simulink model "Lab1"  (R2022b)
settings: Solver=ode45  StartTime=0.0  StopTime=20  RelTol=1e-3
undefined symbols (not defined in the file): T, unicycle
libraries: simulink x2
settings Model: Creator=Musta  LastModifiedBy=Musta

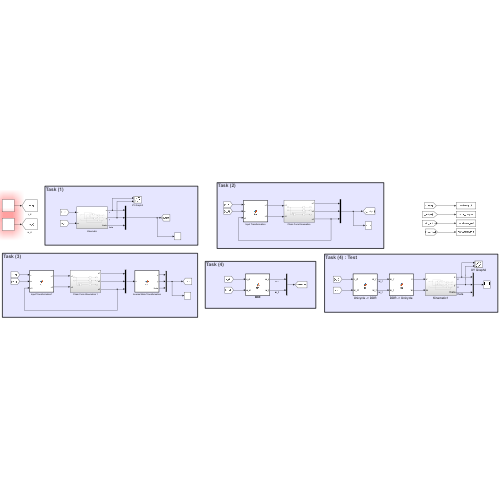
[thumbnail: Simulink's stored preview of the top-level diagram]
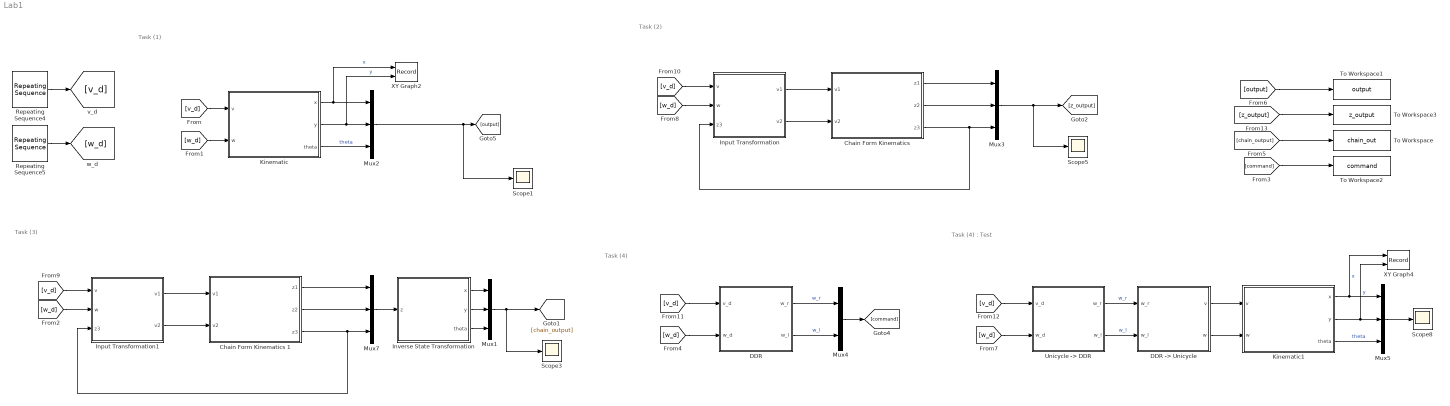
== system Lab1 ==
  note: Task (4) : Test
  note: Task (4)
  note: Task (2)
  note: Task (1)
  note: Task (3)
  " DDR -> Unicycle " : MATLAB Function  TreatAsAtomicUnit=on
  "Chain Form Kinematics " : Subsystem
  Chain Form Kinematics 1 : Subsystem
  DDR : MATLAB Function  TreatAsAtomicUnit=on
  Input Transformation : MATLAB Function  TreatAsAtomicUnit=on
  Input Transformation1 : MATLAB Function  TreatAsAtomicUnit=on
  Inverse State Transformation : MATLAB Function  TreatAsAtomicUnit=on
  Kinematic : Subsystem
  Kinematic1 : Subsystem
  Mux{1..3,5,7} (5 alike) : Mux  Inputs=3
  Mux4 : Mux  Inputs=2
  Repeating Sequence4 : simulink/Sources/Repeating Sequence  rep_seq_t=[0 T/3 2*T/3 T]  rep_seq_y=[0.1 0.1 0.3 0.05]
  Repeating Sequence5 : simulink/Sources/Repeating Sequence  rep_seq_t=[0 T/4 2*T/4 3*T/4 T]  rep_seq_y=[0.0 0.0 0.1 -0.1 0.15]
  Scope{1,3,5,8} (4 alike) : Scope
  To Workspace : ToWorkspace  VariableName=chain_out  SaveFormat=Structure With Time  SampleTime=-1
  To Workspace1 : ToWorkspace  VariableName=output  SaveFormat=Timeseries  SampleTime=-1
  To Workspace2 : ToWorkspace  VariableName=command  SaveFormat=Structure With Time  SampleTime=-1
  To Workspace3 : ToWorkspace  VariableName=z_output  SaveFormat=Structure With Time  SampleTime=-1
  "Unicycle -> DDR" : MATLAB Function  TreatAsAtomicUnit=on
  XY Graph2 : Record  FileSettingsInternal="{\"entries\":[{\"content\":{\"excelSettings\":{\"content\":{},\"type\":\"Streamout.ExcelSettings\"}},\"type\":\"Streamout.FileSettingStorage\",\"uuid\":\"3bdbee54-c759-43d2-8827-5e9ea4f4a11d\"}],\"packageUris\":[\"http://schema.mathworks.com/mf0/streamout_blocks/R2020a\"],\"version\":\"1.0\"}"  Layout=[1 1]  SignalsInternal="{\"entries\":[{\"content\":{\"signals\":[{\"content\":{\"blockPath\":[\"Lab1/XY Graph2\"],\"channel\":[],\"dimensions\":[1],\"domain\":\"Lab1/XY Graph2\",\"lineColor\":\"#a2142f\",\"plots\":[1],\"port\":1,\"sid\":[],\"signalID\":34,\"signalName\":\"x\"},\"type\":\"RecordBlkView.Signal\",\"uuid\":\"4d3c6372-cd81-4779-b9ee-b57c7a1f23b0\"},{\"content\":{\"blockPath\":[\"Lab1/XY Graph2\"],\"channel\":[],\"dimensions\":[1],\"domain\":\"Lab1/XY Graph2\",\"lineColor\":\"#139fff\",\"plots\":[1],\"port\":2,\"sid\":[],\"signalID\":37,\"signalName\":\"y\"},\"type\":\"RecordBlkView.Signal\",\"uuid\":\"7a674121-f9e3-4504-b1cd-7ca841214a66\"}]},\"type\":\"RecordBlkView.InputSignals\",\"uuid\":\"66f41a1e-2d26-4257-ac1b-8d37125b5a9b\"}],\"packageUris\":[\"http://schema.mathworks.com/mf0/streamout_blocks/R2020a\"],\"version\":\"1.0\"}"  VisualizationBindings="{\"xyplotplugin\":{\"info\":[{\"series\":[{\"bindingParametersList\":[{\"parameter\":\"X-Axis\",\"signalID\":34,\"signalName\":\"x\"},{\"parameter\":\"Y-Axis\",\"signalID\":37,\"signalName\":\"y\"}],\"seriesID\":44568}],\"subplotID\":1}]}}"  CompatibilityTag=XY
  XY Graph4 : Record  FileSettingsInternal="{\"entries\":[{\"content\":{\"excelSettings\":{\"content\":{},\"type\":\"Streamout.ExcelSettings\"}},\"type\":\"Streamout.FileSettingStorage\",\"uuid\":\"aad4d6af-3abc-44fb-a7f4-f6db2a127860\"}],\"packageUris\":[\"http://schema.mathworks.com/mf0/streamout_blocks/R2020a\"],\"version\":\"1.0\"}"  Layout=[1 1]  SignalsInternal="{\"entries\":[{\"content\":{\"signals\":[{\"content\":{\"blockPath\":[\"Lab1/XY Graph4\"],\"channel\":[],\"dimensions\":[1],\"domain\":\"Lab1/XY Graph4\",\"lineColor\":\"#a2142f\",\"plots\":[1],\"port\":1,\"sid\":[],\"signalID\":26,\"signalName\":\"x\"},\"type\":\"RecordBlkView.Signal\",\"uuid\":\"5aadf423-cf44-42bb-a75c-07b2a2665d40\"},{\"content\":{\"blockPath\":[\"Lab1/XY Graph4\"],\"channel\":[],\"dimensions\":[1],\"domain\":\"Lab1/XY Graph4\",\"lineColor\":\"#139fff\",\"plots\":[1],\"port\":2,\"sid\":[],\"signalID\":29,\"signalName\":\"y\"},\"type\":\"RecordBlkView.Signal\",\"uuid\":\"69a4f6a6-7bec-4189-9cf2-ac6d9897c812\"}]},\"type\":\"RecordBlkView.InputSignals\",\"uuid\":\"eab3d5d4-c8e6-4073-8c70-e7f334e51194\"}],\"packageUris\":[\"http://schema.mathworks.com/mf0/streamout_blocks/R2020a\"],\"version\":\"1.0\"}"  VisualizationBindings="{\"xyplotplugin\":{\"info\":[{\"series\":[{\"bindingParametersList\":[{\"parameter\":\"X-Axis\",\"signalID\":26,\"signalName\":\"x\"},{\"parameter\":\"Y-Axis\",\"signalID\":29,\"signalName\":\"y\"}],\"seriesID\":23320}],\"subplotID\":1}]}}"  CompatibilityTag=XY
  wires:
  Repeating Sequence4/1 -> [v_d]
  Repeating Sequence5/1 -> [w_d]
  [w_d] -> DDR/2(w_d)
  "Unicycle -> DDR"/2(w_l) -> " DDR -> Unicycle "/2(w_l)  "w_l"
  Input Transformation1/2(v2) -> Chain Form Kinematics 1/2(v2)
  Input Transformation/1(v1) -> "Chain Form Kinematics "/1(v1)
  [w_d] -> "Unicycle -> DDR"/2(w_d)
  Input Transformation1/1(v1) -> Chain Form Kinematics 1/1(v1)
  Chain Form Kinematics 1/2(z2) -> Mux7/2
  [v_d] -> DDR/1(v_d)
  Kinematic1/2(y) -> Mux5/2, XY Graph4/2  "y"
  "Chain Form Kinematics "/2(z2) -> Mux3/2
  "Unicycle -> DDR"/1(w_r) -> " DDR -> Unicycle "/1(w_r)  "w_r"
  Kinematic/3(theta) -> Mux2/3  "theta"
  DDR/2(w_l) -> Mux4/2  "w_l"
  [w_d] -> Input Transformation1/2(w)
  [v_d] -> Input Transformation1/1(v)
  Chain Form Kinematics 1/1(z1) -> Mux7/1
  Kinematic1/1(x) -> Mux5/1, XY Graph4/1  "x"
  Mux5/1 -> Scope8/1
  " DDR -> Unicycle "/1(v) -> Kinematic1/1(v)
  Kinematic1/3(theta) -> Mux5/3  "theta"
  Kinematic/1(x) -> Mux2/1, XY Graph2/1  "x"
  "Chain Form Kinematics "/1(z1) -> Mux3/1
  Kinematic/2(y) -> Mux2/2, XY Graph2/2  "y"
  Chain Form Kinematics 1/3(z3) -> Mux7/3, Input Transformation1/3(z3)
  Input Transformation/2(v2) -> "Chain Form Kinematics "/2(v2)
  [w_d] -> Kinematic/2(w)
  " DDR -> Unicycle "/2(w) -> Kinematic1/2(w)
  Mux3/1 -> [z_output], Scope5/1
  [v_d] -> "Unicycle -> DDR"/1(v_d)
  [v_d] -> Kinematic/1(v)
  Mux7/1 -> Inverse State Transformation/1(z)
  [v_d] -> Input Transformation/1(v)
  [w_d] -> Input Transformation/2(w)
  "Chain Form Kinematics "/3(z3) -> Mux3/3, Input Transformation/3(z3)
  Inverse State Transformation/2(y) -> Mux1/2
  Inverse State Transformation/3(theta) -> Mux1/3
  Mux1/1 -> [chain_output], Scope3/1
  Inverse State Transformation/1(x) -> Mux1/1
  [output] -> To Workspace1/1
  [chain_output] -> To Workspace/1
  [command] -> To Workspace2/1
  Mux2/1 -> Scope1/1, [output]
  Mux4/1 -> [command]
  DDR/1(w_r) -> Mux4/1  "w_r"
  [z_output] -> To Workspace3/1

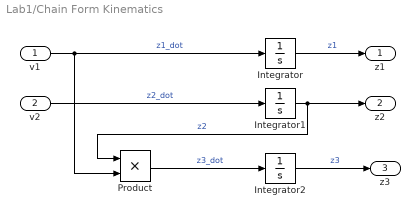
== system Lab1/Chain Form Kinematics  ==
  v1 : Inport
  v2 : Inport  Port=2
  Integrator : Integrator
  Integrator1 : Integrator
  Integrator2 : Integrator
  Product : Product
  z1 : Outport
  z2 : Outport  Port=2
  z3 : Outport  Port=3
  wires:
  v2/1 -> Integrator1/1  "z2_dot"
  v1/1 -> Product/2, Integrator/1  "z1_dot"
  Integrator1/1 -> Product/1, z2/1  "z2"
  Integrator/1 -> z1/1  "z1"
  Product/1 -> Integrator2/1  "z3_dot"
  Integrator2/1 -> z3/1  "z3"

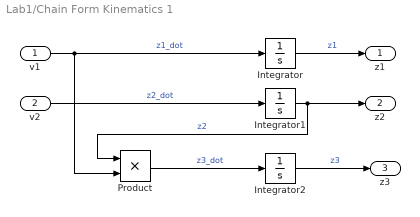
== system Lab1/Chain Form Kinematics 1 ==
  v1 : Inport
  v2 : Inport  Port=2
  Integrator : Integrator
  Integrator1 : Integrator
  Integrator2 : Integrator
  Product : Product
  z1 : Outport
  z2 : Outport  Port=2
  z3 : Outport  Port=3
  wires:
  v2/1 -> Integrator1/1  "z2_dot"
  v1/1 -> Product/2, Integrator/1  "z1_dot"
  Integrator1/1 -> Product/1, z2/1  "z2"
  Integrator/1 -> z1/1  "z1"
  Product/1 -> Integrator2/1  "z3_dot"
  Integrator2/1 -> z3/1  "z3"

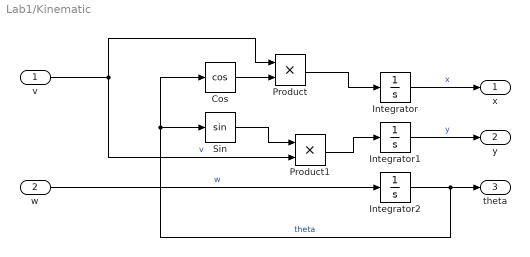
== system Lab1/Kinematic ==
  v : Inport
  w : Inport  Port=2
  Cos : Trigonometry  Operator=cos
  Integrator : Integrator  InitialCondition=unicycle.ic.x
  Integrator1 : Integrator  InitialCondition=unicycle.ic.y
  Integrator2 : Integrator  InitialCondition=unicycle.ic.theta
  Product : Product
  Product1 : Product
  Sin : Trigonometry
  x : Outport
  y : Outport  Port=2
  theta : Outport  Port=3
  wires:
  w/1 -> Integrator2/1  "w"
  Product/1 -> Integrator/1
  v/1 -> Product/1, Product1/2  "v"
  Cos/1 -> Product/2
  Integrator1/1 -> y/1  "y"
  Integrator/1 -> x/1  "x"
  Integrator2/1 -> Cos/1, Sin/1, theta/1  "theta"
  Product1/1 -> Integrator1/1
  Sin/1 -> Product1/1

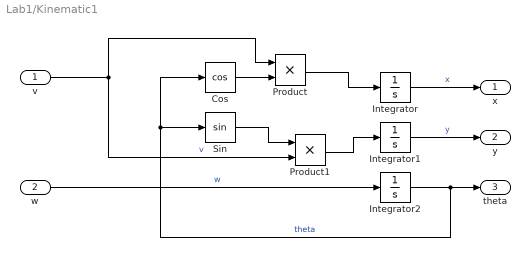
== system Lab1/Kinematic1 ==
  v : Inport
  w : Inport  Port=2
  Cos : Trigonometry  Operator=cos
  Integrator : Integrator  InitialCondition=unicycle.ic.x
  Integrator1 : Integrator  InitialCondition=unicycle.ic.y
  Integrator2 : Integrator  InitialCondition=unicycle.ic.theta
  Product : Product
  Product1 : Product
  Sin : Trigonometry
  x : Outport
  y : Outport  Port=2
  theta : Outport  Port=3
  wires:
  w/1 -> Integrator2/1  "w"
  Product/1 -> Integrator/1
  v/1 -> Product/1, Product1/2  "v"
  Cos/1 -> Product/2
  Integrator1/1 -> y/1  "y"
  Integrator/1 -> x/1  "x"
  Integrator2/1 -> Cos/1, Sin/1, theta/1  "theta"
  Product1/1 -> Integrator1/1
  Sin/1 -> Product1/1

== matlab function Lab1/ DDR -> Unicycle  ==
  data: w_r input; v output; w_l input; w output
function [v, w] = fcn(w_r, w_l)

    %#codegen
    coder.extrinsic('evalin')
    d = 0;                  % Needed in order to set variable class correctly
    r = 0;                  % Needed in order to set variable class correctly
    d = evalin('base','unicycle.d'); % Read value from workspace
    r = evalin('base','unicycle.r'); % Read value from workspace

    v = r*(w_r + w_l)/2; % rad/s
    w = r*(w_r - w_l)/d; % rad/s

end

== matlab function Lab1/DDR ==
  data: v_d input; w_r output; w_d input; w_l output
function [w_r, w_l] = fcn(v_d, w_d)

    %#codegen
    coder.extrinsic('evalin')
    d = 0;                  % Needed in order to set variable class correctly
    r = 0;                  % Needed in order to set variable class correctly
    d = evalin('base','unicycle.d'); % Read value from workspace
    r = evalin('base','unicycle.r'); % Read value from workspace

    w_r = ((2 * v_d) + (w_d * d)) / (2 * r);
    w_l = ((2 * v_d) - (w_d * d)) / (2 * r);

end

== matlab function Lab1/Input Transformation ==
  data: v input; v1 output; w input; v2 output; z3 input
function [v1,v2] = fcn(v,w,z3)

    v1 = w;
    v2 = v - w*z3;

end

== matlab function Lab1/Input Transformation1 ==
  data: v input; v1 output; w input; v2 output; z3 input
function [v1,v2] = fcn(v,w,z3)

    v1 = w;
    v2 = v - w*z3;

end

== matlab function Lab1/Inverse State Transformation ==
  data: z input; x output; y output; theta output
function [x,y,theta] = fcn(z)
    
    theta = z(1);
    T_inv = [0, cos(theta), sin(theta);
             0, sin(theta), -cos(theta);
             1, 0, 0];
    q = T_inv * z;

    x = q(1);
    y = q(2);
    theta = q(3);
    
end

== matlab function Lab1/Unicycle -> DDR ==
  data: v_d input; w_r output; w_d input; w_l output
function [w_r, w_l] = fcn(v_d, w_d)

    %#codegen
    coder.extrinsic('evalin')
    d = 0;                  % Needed in order to set variable class correctly
    r = 0;                  % Needed in order to set variable class correctly
    d = evalin('base','unicycle.d'); % Read value from workspace
    r = evalin('base','unicycle.r'); % Read value from workspace

    w_r = ((2 * v_d) + (w_d * d)) / (2 * r);
    w_l = ((2 * v_d) - (w_d * d)) / (2 * r);

end
